simulink model "ManualDvrCarSim"  (R2016a)
settings: Solver=FixedStepDiscrete  SolverMode=SingleTasking  StartTime=0  StopTime=inf  FixedStep=0.001  RelTol=1e-3  AbsTol=1e-6
PreLoadFcn:
  | PreSettings
InitFcn:
  | set_param(gcs,'StopTime','inf');
undefined symbols (not defined in the file or in its folder): BMotor1, BMotor2, BrkDelayTime, DControlB, Delay1, Delay2, IControlB, JMotor1, JMotor2, PControlB, ratioGearF, ratioGearR, TorqDelayTime, Tstep
libraries: simulink x5, MyLib x3, pil_lib x1
(part 2 of 2)

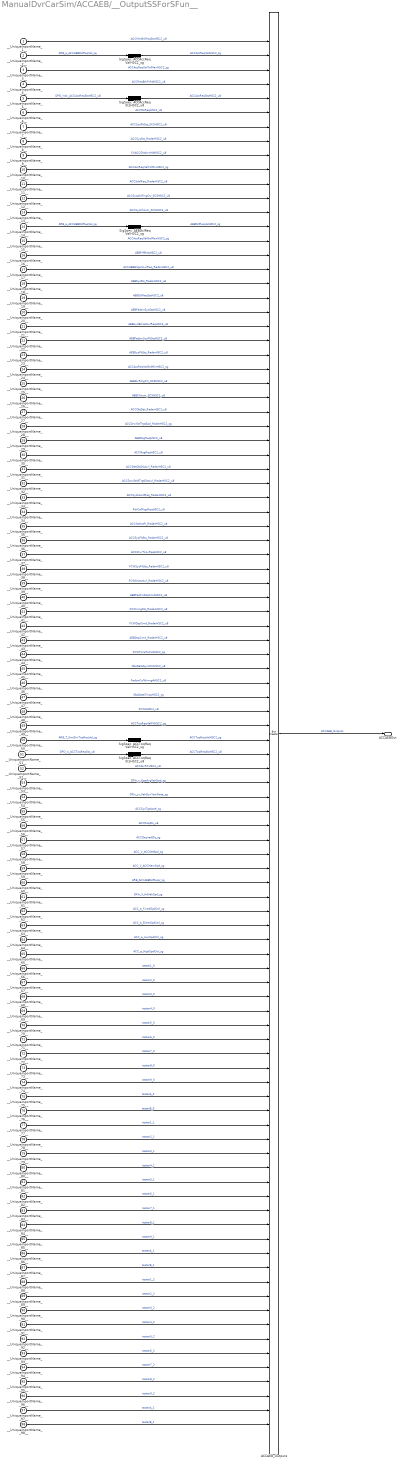
== system ManualDvrCarSim/ACCAEB/__OutputSSForSFun__ ==
  __UniqueInportName__1__ : Inport
  __UniqueInportName__2__ : Inport  Port=2
  __UniqueInportName__3__ : Inport  Port=3
  __UniqueInportName__4__ : Inport  Port=4
  __UniqueInportName__5__ : Inport  Port=5
  __UniqueInportName__6__ : Inport  Port=6
  __UniqueInportName__7__ : Inport  Port=7
  __UniqueInportName__8__ : Inport  Port=8
  __UniqueInportName__9__ : Inport  Port=9
  __UniqueInportName__10__ : Inport  Port=10
  __UniqueInportName__11__ : Inport  Port=11
  __UniqueInportName__12__ : Inport  Port=12
  __UniqueInportName__13__ : Inport  Port=13
  __UniqueInportName__14__ : Inport  Port=14
  __UniqueInportName__15__ : Inport  Port=15
  __UniqueInportName__16__ : Inport  Port=16
  __UniqueInportName__17__ : Inport  Port=17
  __UniqueInportName__18__ : Inport  Port=18
  __UniqueInportName__19__ : Inport  Port=19
  __UniqueInportName__20__ : Inport  Port=20
  __UniqueInportName__21__ : Inport  Port=21
  __UniqueInportName__22__ : Inport  Port=22
  __UniqueInportName__23__ : Inport  Port=23
  __UniqueInportName__24__ : Inport  Port=24
  __UniqueInportName__25__ : Inport  Port=25
  __UniqueInportName__26__ : Inport  Port=26
  __UniqueInportName__27__ : Inport  Port=27
  __UniqueInportName__28__ : Inport  Port=28
  __UniqueInportName__29__ : Inport  Port=29
  __UniqueInportName__30__ : Inport  Port=30
  __UniqueInportName__31__ : Inport  Port=31
  __UniqueInportName__32__ : Inport  Port=32
  __UniqueInportName__33__ : Inport  Port=33
  __UniqueInportName__34__ : Inport  Port=34
  __UniqueInportName__35__ : Inport  Port=35
  __UniqueInportName__36__ : Inport  Port=36
  __UniqueInportName__37__ : Inport  Port=37
  __UniqueInportName__38__ : Inport  Port=38
  __UniqueInportName__39__ : Inport  Port=39
  __UniqueInportName__40__ : Inport  Port=40
  __UniqueInportName__41__ : Inport  Port=41
  __UniqueInportName__42__ : Inport  Port=42
  __UniqueInportName__43__ : Inport  Port=43
  __UniqueInportName__44__ : Inport  Port=44
  __UniqueInportName__45__ : Inport  Port=45
  __UniqueInportName__46__ : Inport  Port=46
  __UniqueInportName__47__ : Inport  Port=47
  __UniqueInportName__48__ : Inport  Port=48
  __UniqueInportName__49__ : Inport  Port=49
  __UniqueInportName__50__ : Inport  Port=50
  __UniqueInportName__51__ : Inport  Port=51
  __UniqueInportName__52__ : Inport  Port=52
  __UniqueInportName__53__ : Inport  Port=53
  __UniqueInportName__54__ : Inport  Port=54
  __UniqueInportName__55__ : Inport  Port=55
  __UniqueInportName__56__ : Inport  Port=56
  __UniqueInportName__57__ : Inport  Port=57
  __UniqueInportName__58__ : Inport  Port=58
  __UniqueInportName__59__ : Inport  Port=59
  __UniqueInportName__60__ : Inport  Port=60
  __UniqueInportName__61__ : Inport  Port=61
  __UniqueInportName__62__ : Inport  Port=62
  __UniqueInportName__63__ : Inport  Port=63
  __UniqueInportName__64__ : Inport  Port=64
  __UniqueInportName__65__ : Inport  Port=65
  __UniqueInportName__66__ : Inport  Port=66
  __UniqueInportName__67__ : Inport  Port=67
  __UniqueInportName__68__ : Inport  Port=68
  __UniqueInportName__69__ : Inport  Port=69
  __UniqueInportName__70__ : Inport  Port=70
  __UniqueInportName__71__ : Inport  Port=71
  __UniqueInportName__72__ : Inport  Port=72
  __UniqueInportName__73__ : Inport  Port=73
  __UniqueInportName__74__ : Inport  Port=74
  __UniqueInportName__75__ : Inport  Port=75
  __UniqueInportName__76__ : Inport  Port=76
  __UniqueInportName__77__ : Inport  Port=77
  __UniqueInportName__78__ : Inport  Port=78
  __UniqueInportName__79__ : Inport  Port=79
  __UniqueInportName__80__ : Inport  Port=80
  __UniqueInportName__81__ : Inport  Port=81
  __UniqueInportName__82__ : Inport  Port=82
  __UniqueInportName__83__ : Inport  Port=83
  __UniqueInportName__84__ : Inport  Port=84
  __UniqueInportName__85__ : Inport  Port=85
  __UniqueInportName__86__ : Inport  Port=86
  __UniqueInportName__87__ : Inport  Port=87
  __UniqueInportName__88__ : Inport  Port=88
  __UniqueInportName__89__ : Inport  Port=89
  __UniqueInportName__90__ : Inport  Port=90
  __UniqueInportName__91__ : Inport  Port=91
  __UniqueInportName__92__ : Inport  Port=92
  __UniqueInportName__93__ : Inport  Port=93
  __UniqueInportName__94__ : Inport  Port=94
  __UniqueInportName__95__ : Inport  Port=95
  __UniqueInportName__96__ : Inport  Port=96
  __UniqueInportName__97__ : Inport  Port=97
  __UniqueInportName__98__ : Inport  Port=98
  ACCAEB_Outputs : BusCreator  Inputs=98
  SigSpec_ACCAccReqStsHSC2_u8 : Demux  Outputs=1
  SigSpec_ACCAccReqValHSC2_sg : Demux  Outputs=1
  SigSpec_ACCToqReqStsHSC2_u8 : Demux  Outputs=1
  SigSpec_ACCToqReqValHSC2_sg : Demux  Outputs=1
  SigSpec_AEBDclReqValHSC2_sg : Demux  Outputs=1
  ACCAEBOut : Outport
  wires:
  __UniqueInportName__2__/1 -> SigSpec_ACCAccReqValHSC2_sg/1  "ARB_a_ACCAEBDclReqVal_sg"
  __UniqueInportName__5__/1 -> SigSpec_ACCAccReqStsHSC2_u8/1  "DPO_indx_ACCAccReqStsHSC2_u8"
  __UniqueInportName__14__/1 -> SigSpec_AEBDclReqValHSC2_sg/1  "ARB_a_ACCAEBDclReqVal_sg"
  __UniqueInportName__50__/1 -> SigSpec_ACCToqReqValHSC2_sg/1  "ARB_T_SmtDrvToqReqVal_sg"
  __UniqueInportName__51__/1 -> SigSpec_ACCToqReqStsHSC2_u8/1  "DPO_is_ACCToqReqSts_u8"
  __UniqueInportName__1__/1 -> ACCAEB_Outputs/1  "ACCMinBrkReqStsHSC2_u8"
  SigSpec_ACCAccReqValHSC2_sg/1 -> ACCAEB_Outputs/2  "ACCAccReqValHSC2_sg"
  __UniqueInportName__3__/1 -> ACCAEB_Outputs/3  "ACCAccReqValTolMaxHSC2_sg"
  __UniqueInportName__4__/1 -> ACCAEB_Outputs/4  "ACCReqBrkPrfrdHSC2_u8"
  SigSpec_ACCAccReqStsHSC2_u8/1 -> ACCAEB_Outputs/5  "ACCAccReqStsHSC2_u8"
  __UniqueInportName__6__/1 -> ACCAEB_Outputs/6  "ACCGoReqHSC2_u8"
  __UniqueInportName__7__/1 -> ACCAEB_Outputs/7  "ACCSysFltSts_SCSHSC2_u8"
  __UniqueInportName__8__/1 -> ACCAEB_Outputs/8  "ACCSysSts_RadarHSC2_u8"
  __UniqueInportName__9__/1 -> ACCAEB_Outputs/9  "ChACCShtdwnMdHSC2_u8"
  __UniqueInportName__10__/1 -> ACCAEB_Outputs/10  "ACCAccReqValTolMinHSC2_sg"
  __UniqueInportName__11__/1 -> ACCAEB_Outputs/11  "ACCSdslReq_RadarHSC2_u8"
  __UniqueInportName__12__/1 -> ACCAEB_Outputs/12  "ACCSysAlvRlngCtr_SCSHSC2_u8"
  __UniqueInportName__13__/1 -> ACCAEB_Outputs/13  "ACCSysChksm_SCSHSC2_u8"
  SigSpec_AEBDclReqValHSC2_sg/1 -> ACCAEB_Outputs/14  "AEBDclReqValHSC2_sg"
  __UniqueInportName__15__/1 -> ACCAEB_Outputs/15  "ACCAccReqValGrdMaxHSC2_sg"
  __UniqueInportName__16__/1 -> ACCAEB_Outputs/16  "AEBPrflReqHSC2_u8"
  __UniqueInportName__17__/1 -> ACCAEB_Outputs/17  "ACCAEBBrkJerkLvlReq_RadarHSC2_u8"
  __UniqueInportName__18__/1 -> ACCAEB_Outputs/18  "AEBSysSts_RadarHSC2_u8"
  __UniqueInportName__19__/1 -> ACCAEB_Outputs/19  "AEBDclReqStsHSC2_u8"
  __UniqueInportName__20__/1 -> ACCAEB_Outputs/20  "AEBPedtrnSysStsHSC2_u8"
  __UniqueInportName__21__/1 -> ACCAEB_Outputs/21  "AEBHydBrkAstLvlReqHSC2_u8"
  __UniqueInportName__22__/1 -> ACCAEB_Outputs/22  "AEBPedtrnSysFltStsHSC2_u8"
  __UniqueInportName__23__/1 -> ACCAEB_Outputs/23  "AEBSysFltSts_RadarHSC2_u8"
  __UniqueInportName__24__/1 -> ACCAEB_Outputs/24  "ACCAccReqValGrdMinHSC2_sg"
  __UniqueInportName__25__/1 -> ACCAEB_Outputs/25  "AEBAlvRlngCtr_SCSHSC2_u8"
  __UniqueInportName__26__/1 -> ACCAEB_Outputs/26  "AEBChksm_SCSHSC2_u8"
  __UniqueInportName__27__/1 -> ACCAEB_Outputs/27  "ACCObjDet_RadarHSC2_u8"
  __UniqueInportName__28__/1 -> ACCAEB_Outputs/28  "ACCDrvrSelTrgtSpd_RadarHSC2_sg"
  __UniqueInportName__29__/1 -> ACCAEB_Outputs/29  "AEBMsgReqHSC2_u8"
  __UniqueInportName__30__/1 -> ACCAEB_Outputs/30  "ACCMsgReqHSC2_u8"
  __UniqueInportName__31__/1 -> ACCAEB_Outputs/31  "ACCDetObjDistLvl_RadarHSC2_u8"
  __UniqueInportName__32__/1 -> ACCAEB_Outputs/32  "ACCDrvrSeldTrgtDistLvl_RadarHSC2_u8"
  __UniqueInportName__33__/1 -> ACCAEB_Outputs/33  "ACCSysCanclReq_RadarHSC2_u8"
  __UniqueInportName__34__/1 -> ACCAEB_Outputs/34  "RdrCalPrgsReqHSC2_u8"
  __UniqueInportName__35__/1 -> ACCAEB_Outputs/35  "ACCGoNotfr_RadarHSC2_u8"
  __UniqueInportName__36__/1 -> ACCAEB_Outputs/36  "ACCSysFltSts_RadarHSC2_u8"
  __UniqueInportName__37__/1 -> ACCAEB_Outputs/37  "ACCDrvrTkovReqHSC2_u8"
  __UniqueInportName__38__/1 -> ACCAEB_Outputs/38  "FCWSysFltSts_RadarHSC2_u8"
  __UniqueInportName__39__/1 -> ACCAEB_Outputs/39  "FCWSnstvtLvl_RadarHSC2_u8"
  __UniqueInportName__40__/1 -> ACCAEB_Outputs/40  "AEBPedtrnDspCmdHSC2_u8"
  __UniqueInportName__41__/1 -> ACCAEB_Outputs/41  "FCWrnngSts_RadarHSC2_u8"
  __UniqueInportName__42__/1 -> ACCAEB_Outputs/42  "FCWDspCmd_RadarHSC2_u8"
  __UniqueInportName__43__/1 -> ACCAEB_Outputs/43  "AEBDspCmd_RadarHSC2_u8"
  __UniqueInportName__44__/1 -> ACCAEB_Outputs/44  "FCWTimeToColHSC2_sg"
  __UniqueInportName__45__/1 -> ACCAEB_Outputs/45  "ObsDataSyncCtrHSC2_u8"
  __UniqueInportName__46__/1 -> ACCAEB_Outputs/46  "PedtrnColWrnngAHSC2_u8"
  __UniqueInportName__47__/1 -> ACCAEB_Outputs/47  "ObsDataTmspHSC2_sg"
  __UniqueInportName__48__/1 -> ACCAEB_Outputs/48  "FCWAHSC2_u8"
  __UniqueInportName__49__/1 -> ACCAEB_Outputs/49  "ACCToqReqValPVHSC2_sg"
  SigSpec_ACCToqReqValHSC2_sg/1 -> ACCAEB_Outputs/50  "ACCToqReqValHSC2_sg"
  SigSpec_ACCToqReqStsHSC2_u8/1 -> ACCAEB_Outputs/51  "ACCToqReqStsHSC2_u8"
  __UniqueInportName__52__/1 -> ACCAEB_Outputs/52  "ACCAlvRCHSC2_u8"
  __UniqueInportName__53__/1 -> ACCAEB_Outputs/53  "DFIn_v_EgoAvgVehSpd_sg"
  __UniqueInportName__54__/1 -> ACCAEB_Outputs/54  "DFIn_yr_VehDynYawRate_sg"
  __UniqueInportName__55__/1 -> ACCAEB_Outputs/55  "ACCSysTgtAccel_sg"
  __UniqueInportName__56__/1 -> ACCAEB_Outputs/56  "ACCReqSts_u8"
  __UniqueInportName__57__/1 -> ACCAEB_Outputs/57  "ACCDesiredDis_sg"
  __UniqueInportName__58__/1 -> ACCAEB_Outputs/58  "ACC_V_ACCSetSpd_sg"
  __UniqueInportName__59__/1 -> ACCAEB_Outputs/59  "ACC_V_ACCMemSpd_sg"
  __UniqueInportName__60__/1 -> ACCAEB_Outputs/60  "ARB_ACCAEBDclReqV_sg"
  __UniqueInportName__61__/1 -> ACCAEB_Outputs/61  "DFIn_V_HdVehSpd_sg"
  __UniqueInportName__62__/1 -> ACCAEB_Outputs/62  "ACC_a_FixedSpdCtrl_sg"
  __UniqueInportName__63__/1 -> ACCAEB_Outputs/63  "ACC_a_EmerSpdCtrl_sg"
  __UniqueInportName__64__/1 -> ACCAEB_Outputs/64  "ACC_a_LowSpdCtrl_sg"
  __UniqueInportName__65__/1 -> ACCAEB_Outputs/65  "ACC_a_HighSpdCtrl_sg"
  __UniqueInportName__66__/1 -> ACCAEB_Outputs/66  "tester1_0"
  __UniqueInportName__67__/1 -> ACCAEB_Outputs/67  "tester2_0"
  __UniqueInportName__68__/1 -> ACCAEB_Outputs/68  "tester3_0"
  __UniqueInportName__69__/1 -> ACCAEB_Outputs/69  "tester4_0"
  __UniqueInportName__70__/1 -> ACCAEB_Outputs/70  "tester5_0"
  __UniqueInportName__71__/1 -> ACCAEB_Outputs/71  "tester6_0"
  __UniqueInportName__72__/1 -> ACCAEB_Outputs/72  "tester7_0"
  __UniqueInportName__73__/1 -> ACCAEB_Outputs/73  "tester8_0"
  __UniqueInportName__74__/1 -> ACCAEB_Outputs/74  "tester9_0"
  __UniqueInportName__75__/1 -> ACCAEB_Outputs/75  "testerA_0"
  __UniqueInportName__76__/1 -> ACCAEB_Outputs/76  "testerB_0"
  __UniqueInportName__77__/1 -> ACCAEB_Outputs/77  "tester1_1"
  __UniqueInportName__78__/1 -> ACCAEB_Outputs/78  "tester2_1"
  __UniqueInportName__79__/1 -> ACCAEB_Outputs/79  "tester3_1"
  __UniqueInportName__80__/1 -> ACCAEB_Outputs/80  "tester4_1"
  __UniqueInportName__81__/1 -> ACCAEB_Outputs/81  "tester5_1"
  __UniqueInportName__82__/1 -> ACCAEB_Outputs/82  "tester6_1"
  __UniqueInportName__83__/1 -> ACCAEB_Outputs/83  "tester7_1"
  __UniqueInportName__84__/1 -> ACCAEB_Outputs/84  "tester8_1"
  __UniqueInportName__85__/1 -> ACCAEB_Outputs/85  "tester9_1"
  __UniqueInportName__86__/1 -> ACCAEB_Outputs/86  "testerA_1"
  __UniqueInportName__87__/1 -> ACCAEB_Outputs/87  "testerB_1"
  __UniqueInportName__88__/1 -> ACCAEB_Outputs/88  "tester1_2"
  __UniqueInportName__89__/1 -> ACCAEB_Outputs/89  "tester2_2"
  __UniqueInportName__90__/1 -> ACCAEB_Outputs/90  "tester3_2"
  __UniqueInportName__91__/1 -> ACCAEB_Outputs/91  "tester4_2"
  __UniqueInportName__92__/1 -> ACCAEB_Outputs/92  "tester5_2"
  __UniqueInportName__93__/1 -> ACCAEB_Outputs/93  "tester6_2"
  __UniqueInportName__94__/1 -> ACCAEB_Outputs/94  "tester7_2"
  __UniqueInportName__95__/1 -> ACCAEB_Outputs/95  "tester8_2"
  __UniqueInportName__96__/1 -> ACCAEB_Outputs/96  "tester9_2"
  __UniqueInportName__97__/1 -> ACCAEB_Outputs/97  "testerA_2"
  __UniqueInportName__98__/1 -> ACCAEB_Outputs/98  "testerB_2"
  ACCAEB_Outputs/1 -> ACCAEBOut/1  "ACCAEB_Outputs"

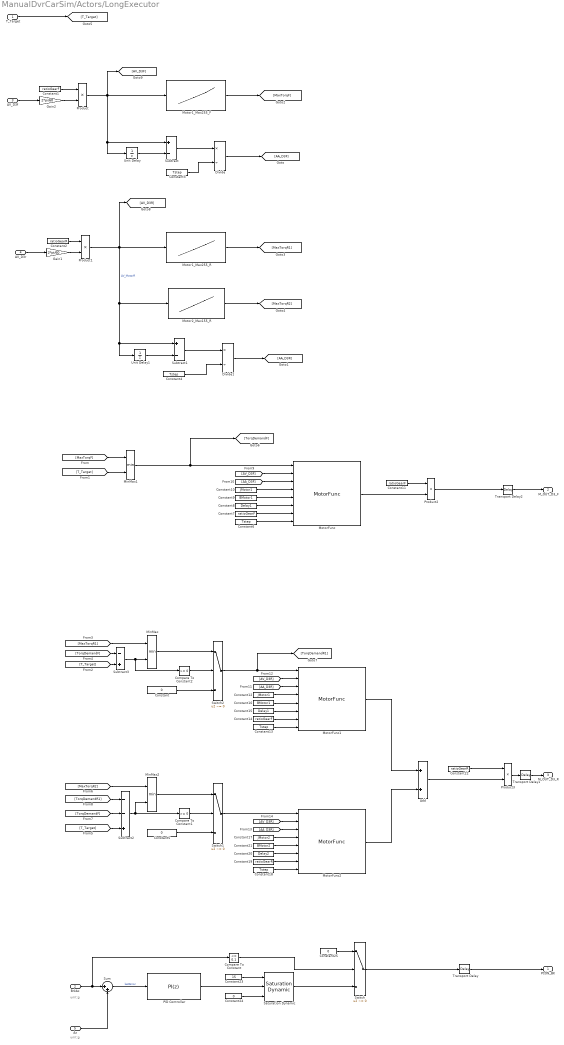
== system ManualDvrCarSim/Actors/LongExecutor ==
  note: unit:g
  note: unit:g
  T_Target : Inport
  BrkAx : Inport  Port=2
  AV_D3f : Inport  Port=3
  AV_D3r : Inport  Port=4
  Ax : Inport  Port=5
  Add : Sum
  Compare To Constant : simulink/Logic and Bit Operations/Compare To Constant  relop=<=  const=0.1  OutDataTypeStr=boolean
  Compare To Constant1 : simulink/Logic and Bit Operations/Compare To Constant  relop=>=  const=0  OutDataTypeStr=boolean
  Compare To Constant2 : simulink/Logic and Bit Operations/Compare To Constant  relop=>=  const=0  OutDataTypeStr=boolean
  Constant{,5,24..25} (4 alike) : Constant  Value=0
  Constant{1,7,11,14} (4 alike) : Constant  Value=ratioGearF
  Constant10 : Constant  Value=JMotor1
  Constant12 : Constant  Value=JMotor1
  Constant{3..4,6,13,18} (5 alike) : Constant  Value=Tstep
  Constant15 : Constant  Value=Delay1
  Constant16 : Constant  Value=BMotor1
  Constant17 : Constant  Value=JMotor2
  Constant19 : Constant  Value=ratioGearR
  Constant2 : Constant  Value=ratioGearR
  Constant20 : Constant  Value=Delay2
  Constant21 : Constant  Value=BMotor2
  Constant22 : Constant  Value=ratioGearR
  Constant23 : Constant  Value=15
  Constant8 : Constant  Value=Delay1
  Constant9 : Constant  Value=BMotor1
  Divide : Product  Inputs=*/
  Divide1 : Product  Inputs=*/
  Gain1 : Gain  Gain=2*pi/60
  Gain2 : Gain  Gain=2*pi/60
  MinMax : MinMax  Inputs=2
  MinMax1 : MinMax  Inputs=2
  MinMax2 : MinMax  Inputs=2
  Motor1_Max255_F : Lookup_n-D  NumberOfTableDimensions=1  BreakpointsForDimension1="[-1047.2,-942.48,-837.76,-733.04,-628.32,-523.6,-418.88,-314.16,-209.44,-104.72,-52.36,-0.1,0,0.1,52.36,104.72,209.44,314.16,418.88,523.6\t628.32,733.04,837.76,942.48,1047.2]"  Table=[-67,-79,-92,-108,-130,-159,-204,-255,-255,-255,-255,-255,255,255,255,255,255,255,204,159,130,108,92,79,67]  InternalRulePriority=Speed  RndMeth=Simplest  InputSameDT=on
  Motor1_Max255_R : Lookup_n-D  NumberOfTableDimensions=1  BreakpointsForDimension1="[-1047.2,-942.48,-837.76,-733.04,-628.32,-523.6,-418.88,-314.16,-209.44,-104.72,-52.36,-0.1,0,0.1,52.36,104.72,209.44,314.16,418.88,523.6\t628.32,733.04,837.76,942.48,1047.2]"  Table=[-67,-79,-92,-108,-130,-159,-204,-255,-255,-255,-255,-255,255,255,255,255,255,255,204,159,130,108,92,79,67]  InternalRulePriority=Speed  RndMeth=Simplest  InputSameDT=on
  Motor2_Max155_R : Lookup_n-D  NumberOfTableDimensions=1  BreakpointsForDimension1="[-1047.2,-942.48,-837.76,-733.04,-628.32,-523.6,-418.88,-314.16,-209.44,-104.72,-52.36,-0.1,0,0.1,52.36,104.72,209.44,314.16,418.88,523.6\t628.32,733.04,837.76,942.48,1047.2]"  Table="[-46.6,-52.3,-58.93,-69,-82.5,-99.5,-124.5,-155,-155,-155\t,-155,-155,155,155,155,155,155,155,124.5,99.5,82.5,69,58.93,52.3,46.6]"  InternalRulePriority=Speed  RndMeth=Simplest  InputSameDT=on
  MotorFunc : MyLib/MotorFunc
  MotorFunc1 : MyLib/MotorFunc
  MotorFunc2 : MyLib/MotorFunc
  PID Controller : simulink/Continuous/PID Controller  Controller=PI  TimeDomain=Discrete-time  SampleTime=0.001  IntegratorMethod=Forward Euler  FilterMethod=Forward Euler  Form=Parallel  UseFilter=on  ControllerParametersSource=internal  P=PControlB  I=IControlB  D=DControlB  N=100  InitialConditionSource=internal  InitialConditionForIntegrator=0  InitialConditionForFilter=0  ExternalReset=none  LimitOutput=off  UpperSaturationLimit=inf  LowerSaturationLimit=-inf  LinearizeAsGain=on  AntiWindupMode=none  Kb=1  TrackingMode=off  Kt=1  PParamMin=[]  PParamMax=[]  IParamMin=[]  IParamMax=[]  DParamMin=[]  DParamMax=[]  NParamMin=[]  NParamMax=[]  KbParamMin=[]  KbParamMax=[]  KtParamMin=[]  KtParamMax=[]  POutMin=[]  POutMax=[]  IOutMin=[]  IOutMax=[]  DOutMin=[]  DOutMax=[]  NOutMin=[]  NOutMax=[]  KbOutMin=[]  KbOutMax=[]  KtOutMin=[]  KtOutMax=[]  IntegratorOutMin=[]  IntegratorOutMax=[]  FilterOutMin=[]  FilterOutMax=[]  SumOutMin=[]  SumOutMax=[]  SumI1OutMin=[]  SumI1OutMax=[]  SumI2OutMin=[]  SumI2OutMax=[]  SumI3OutMin=[]  SumI3OutMax=[]  SumDOutMin=[]  SumDOutMax=[]  SaturationOutMin=[]  SaturationOutMax=[]  IntegratorContinuousStateAttributes=''  IntegratorStateMustResolveToSignalObject=off  IntegratorRTWStateStorageClass=Auto  FilterContinuousStateAttributes=''  FilterStateMustResolveToSignalObject=off  FilterRTWStateStorageClass=Auto  DifferentiatorICPrevScaledInput=0  DifferentiatorOutMin=[]  DifferentiatorOutMax=[]
  Product{,1..3} (4 alike) : Product
  Saturation Dynamic : simulink/Discontinuities/Saturation Dynamic  OutMin=[]  OutMax=[]  OutDataTypeStr=Inherit: Same as second input  OutDataType=fixdt(1, 16)  OutScaling=2^-10  DoSatur=off
  Subtract : Sum  Inputs=+-
  Subtract1 : Sum  Inputs=+-
  Subtract2 : Sum  Inputs=--+
  Subtract3 : Sum  Inputs=-+
  Sum : Sum  Inputs=|++
  Switch : Switch  Criteria=u2 ~= 0
  Switch1 : Switch  Criteria=u2 ~= 0
  Switch2 : Switch  Criteria=u2 ~= 0
  Transport Delay : TransportDelay  DelayTime=BrkDelayTime
  Transport Delay1 : TransportDelay  DelayTime=TorqDelayTime
  Transport Delay2 : TransportDelay  DelayTime=TorqDelayTime
  Unit Delay : UnitDelay  SampleTime=-1
  Unit Delay1 : UnitDelay  SampleTime=-1
  PCON_BK : Outport
  M_OUT_D3_F : Outport  Port=2
  M_OUT_D3_R : Outport  Port=3
  wires:
  AV_D3f/1 -> Gain2/1
  Constant1/1 -> Product/1
  AV_D3r/1 -> Gain1/1
  Constant2/1 -> Product1/1
  Product/1 -> [AV_D3F], Unit Delay/1, Subtract/1, Motor1_Max255_F/1
  Unit Delay/1 -> Subtract/2
  Subtract/1 -> Divide/1
  Constant3/1 -> Divide/2
  Motor1_Max255_F/1 -> [MaxTorqF]
  Product1/1 -> [AV_D3R], Unit Delay1/1, Subtract1/1, Motor2_Max155_R/1, Motor1_Max255_R/1  "AV_MotorR"
  Divide/1 -> [AA_D3F]
  Unit Delay1/1 -> Subtract1/2
  Subtract1/1 -> Divide1/1
  Constant4/1 -> Divide1/2
  Divide1/1 -> [AA_D3R]
  Motor1_Max255_R/1 -> [MaxTorqR1]
  Motor2_Max155_R/1 -> [MaxTorqR2]
  T_Target/1 -> [T_Target]
  [MaxTorqF] -> MinMax1/1
  [T_Target] -> MinMax1/2
  MinMax1/1 -> MotorFunc/1, [TorqDemandF]
  [TorqDemandF] -> Subtract3/1
  [T_Target] -> Subtract3/2
  Subtract3/1 -> Compare To Constant2/1, MinMax/2
  [MaxTorqR1] -> MinMax/1
  MinMax/1 -> Switch2/1
  Compare To Constant2/1 -> Switch2/2
  Constant/1 -> Switch2/3
  [TorqDemandF] -> Subtract2/2
  [T_Target] -> Subtract2/3
  Subtract2/1 -> MinMax2/2, Compare To Constant1/1
  [MaxTorqR2] -> MinMax2/1
  MinMax2/1 -> Switch1/1
  Compare To Constant1/1 -> Switch1/2
  Constant5/1 -> Switch1/3
  [TorqDemandR1] -> Subtract2/1
  Constant6/1 -> MotorFunc/8
  Constant7/1 -> MotorFunc/7
  Constant8/1 -> MotorFunc/6
  Constant9/1 -> MotorFunc/5
  Constant10/1 -> MotorFunc/4
  [AV_D3F] -> MotorFunc/2
  [AA_D3F] -> MotorFunc/3
  Constant11/1 -> Product2/1
  Product2/1 -> Transport Delay2/1
  Switch2/1 -> MotorFunc1/1, [TorqDemandR1]
  [AV_D3R] -> MotorFunc1/2
  [AA_D3R] -> MotorFunc1/3
  Constant12/1 -> MotorFunc1/4
  Constant16/1 -> MotorFunc1/5
  Constant15/1 -> MotorFunc1/6
  Constant14/1 -> MotorFunc1/7
  Constant13/1 -> MotorFunc1/8
  Switch1/1 -> MotorFunc2/1
  [AV_D3R] -> MotorFunc2/2
  [AA_D3R] -> MotorFunc2/3
  Constant17/1 -> MotorFunc2/4
  Constant21/1 -> MotorFunc2/5
  Constant20/1 -> MotorFunc2/6
  Constant19/1 -> MotorFunc2/7
  Constant18/1 -> MotorFunc2/8
  Constant22/1 -> Product3/1
  Product3/1 -> Transport Delay1/1
  Add/1 -> Product3/2
  MotorFunc1/1 -> Add/1
  MotorFunc2/1 -> Add/2
  Ax/1 -> Sum/2
  BrkAx/1 -> Compare To Constant/1, Sum/1
  Sum/1 -> PID Controller/1  "lastError"
  Constant23/1 -> Saturation Dynamic/1
  Constant24/1 -> Saturation Dynamic/3
  Saturation Dynamic/1 -> Switch/3
  Compare To Constant/1 -> Switch/2
  Constant25/1 -> Switch/1
  Switch/1 -> Transport Delay/1
  Gain1/1 -> Product1/2
  Gain2/1 -> Product/2
  Transport Delay/1 -> PCON_BK/1
  Transport Delay1/1 -> M_OUT_D3_R/1
  Transport Delay2/1 -> M_OUT_D3_F/1
  MotorFunc/1 -> Product2/2
  PID Controller/1 -> Saturation Dynamic/2

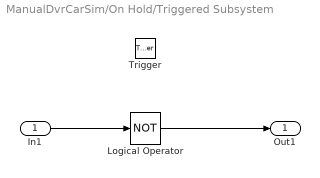
== system ManualDvrCarSim/On Hold/Triggered Subsystem ==
  In1 : Inport
  Trigger : TriggerPort  VariantControl=Variant
  Logical Operator : Logic  Operator=NOT  AllPortsSameDT=off  OutDataTypeStr=boolean
  Out1 : Outport
  wires:
  In1/1 -> Logical Operator/1
  Logical Operator/1 -> Out1/1
